simulink model "GetStatus"  (R2024a)
settings: Solver=FixedStepAuto  StartTime=0.0  StopTime=10.0  RelTol=1e-3
libraries: autosarlibdem x2
settings Model: Creator=buiqu  LastModifiedBy=buiqu
settings OptimizationCC: DefaultParameterBehavior=Inlined  EnhancedBackFolding=on  PassReuseOutputArgsAs=Individual arguments  ZeroExternalMemoryAtStartup=off  ZeroInternalMemoryAtStartup=off  OptimizeBlockOrder=speed  DifferentSizesBufferReuse=on  OptimizationCustomize=off  EfficientTunableParamExpr=on
settings DebuggingCC: ParameterTunabilityLossMsg=error
settings SFSimCC: MATLABDynamicMemAlloc=off
settings RTWCC: Description=AUTOSAR  SystemTargetFile=autosar.tlc  GenCodeOnly=on  TemplateMakefile=ert_default_tmf  DataTypeReplacement=CDataTypesFixedWidth
settings CodeAppCC: ForceParamTrailComments=on  IgnoreCustomStorageClasses=off  OperatorAnnotations=on  SimulinkDataObjDesc=on  SFDataObjDesc=on  InsertBlockDesc=on
settings STFCustomTargetCC: MultiwordLength=256  ParMdlRefBuildCompliant=on  CompOptLevelCompliant=on  IncludeMdlTerminateFcn=off  CombineOutputUpdateFcns=on  SuppressErrorStatus=on  ERTCustomFileBanners=on  SupportNonFinite=off  SupportComplex=off  SupportContinuousTime=off  SupportNonInlinedSFcns=off  RemoveResetFunc=on  MATLABClassNameForMDSCustomization=Simulink.SoftwareTarget.ERTCustomization  AutosarCompliant=on  GRTInterface=off  LookupTableObjectStructAxisOrder=2,1,3,4,...  LUTObjectStructOrderEvenSpacing=Size,Table,Breakpoints  SystemTargetFile=autosar.tlc
settings ERTTargetCC: TargetLangStandard=C99 (ISO)  ConcurrentExecutionCompliant=off  IncludeMdlTerminateFcn=off  SuppressErrorStatus=on  SupportNonFinite=off  SupportComplex=off  ModelStepFunctionPrototypeControlCompliant=off  CPPClassGenCompliant=off  AutosarCompliant=on  LookupTableObjectStructAxisOrder=2,1,3,4,...  LUTObjectStructOrderEvenSpacing=Size,Table,Breakpoints  InlinedParameterPlacement=NonHierarchical  ERTCustomFileTemplate=example_file_process.tlc  BooleanTrueId=TRUE  BooleanFalseId=FALSE

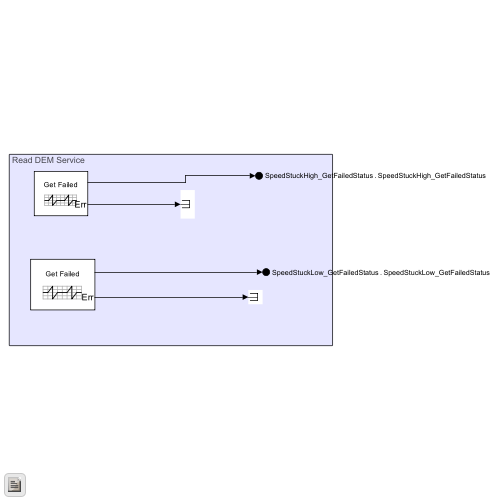
[thumbnail: Simulink's stored preview of the top-level diagram]
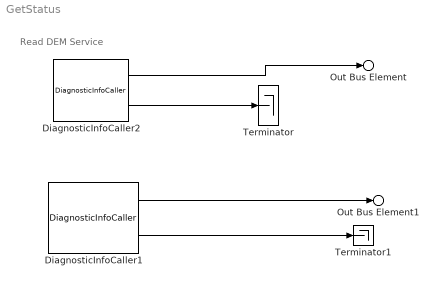
== system GetStatus ==
  note: Read DEM Service
  DiagnosticInfoCaller1 : autosarlibdem/DiagnosticInfoCaller  PortName=SpeedStuckLow  Operation=GetEventFailed  st=-1  ServiceImpl=autosar.bsw.DemDiagnosticInfo  SyncToSchema=off
  DiagnosticInfoCaller2 : autosarlibdem/DiagnosticInfoCaller  PortName=SpeedStuckHigh  Operation=GetEventFailed  st=-1  ServiceImpl=autosar.bsw.DemDiagnosticInfo  SyncToSchema=off
  Terminator : Terminator
  Terminator1 : Terminator
  Out Bus Element : Outport  PortName=SpeedStuckHigh_GetFailedStatus  Element=SpeedStuckHigh_GetFailedStatus
  Out Bus Element1 : Outport  Port=2  PortName=SpeedStuckLow_GetFailedStatus  Element=SpeedStuckLow_GetFailedStatus
  wires:
  DiagnosticInfoCaller1/2 -> Terminator1/1
  DiagnosticInfoCaller2/2 -> Terminator/1
  DiagnosticInfoCaller2/1 -> Out Bus Element/1
  DiagnosticInfoCaller1/1 -> Out Bus Element1/1
